simulink model "ID_Simulator"  (R2017b)
settings: Solver=VariableStepAuto  StartTime=0  StopTime=12  FixedStep=0.0005  EnableMultiTasking=on
InitFcn:
  | isSim = 1;
  | PreFunctions.CustomInitFcn;
  | PreFunctions.simulationInitFcn
values from neighbouring files (symbols this model uses):
  s = 0    [state_estimation.m]
undefined symbols (not defined in the file or in its folder): DiagnosticCodes, fcut_velocity_joint, GaitLibrary, motorPositions, motorVelocities, pelvisPosition, pelvisVelocity, UserParams, X, Y, Z
libraries: sm_lib x112, nesl_utility x20, ComponentLibrary x15, Contact_Forces_Lib x4, slrtlib x1, simulink x1, func_block_library x1
(part 1 of 5)
settings Model: Creator=case  LastModifiedBy=guoro
settings SolverCC: ZeroCrossControl=DisableAll  InsertRTBMode=Always
settings DataIOCC: SaveFormat=Array  SaveOutput=off  SaveState=on  DSMLogging=off
settings OptimizationCC: DefaultParameterBehavior=Inlined  UseFloatMulNetSlope=on  InlineInvariantSignals=on  EfficientFloat2IntCast=on  LifeSpan=inf  SimCompilerOptimization=on  AccelVerboseBuild=on
settings DebuggingCC: ReadBeforeWriteMsg=DisableAll  WriteAfterWriteMsg=DisableAll  WriteAfterReadMsg=DisableAll  ParameterUnderflowMsg=error  ParameterTunabilityLossMsg=error  UniqueDataStoreMsg=error  AllowSymbolicDim=off  StrictBusMsg=ErrorOnBusTreatedAsVector  SFUnexpectedBacktrackingDiag=warning  SFNoUnconditionalDefaultTransitionDiag=warning  SFExecutionAtInitializationDiag=none
settings HardwareCC: TargetBitPerPointer=64  TargetBitPerSizeT=64  TargetBitPerPtrDiffT=64  TargetLongLongMode=on  TargetIntDivRoundTo=Zero  TargetEndianess=LittleEndian  TargetWordSize=64  TargetHWDeviceType=MATLAB Host  ProdEqTarget=off
settings ModelReferenceCC: EnableParallelModelReferenceBuilds=on  ModelReferenceNumInstancesAllowed=Zero  ModelReferenceMinAlgLoopOccurrences=on  PropagateSignalLabelsOutOfModel=off
settings SFSimCC: SimUserIncludeDirs=gen\kin\src
settings SFSimCC: SimUserSources=|
  | ComPosition_src.c
  | ComVelocity_src.c
  | J_LeftToeBottomBack_src.c
  | J_LeftToeBottomFront_src.c
  | J_LeftToeBottom_src.c
  | J_LeftToeJoint_src.c
  | J_RightToeBottomBack_src.c
  | J_RightToeBottomFront_src.c
  | J_RightToeBottom_src.c
  | J_RightToeJoint_src.c
  | LeftToeBottomBack_src.c
  | LeftToeBottomFront_src.c
  | LeftToeBottom_src.c
  | LeftToeJoint_src.c
  | RightToeBottomBack_src.c
  | RightToeBottomFront_src.c
  | RightToeBottom_src.c
  | RightToeJoint_src.c
settings RTWCC: Description=Generic Real-Time Target  RTWUseSimCustomCode=on  CustomInclude=gen\kin\src  BuildConfiguration=Faster Runs  CheckMdlBeforeBuild=Warning
settings RTWCC: CustomSource=|
  | ComPosition_src.c
  | ComVelocity_src.c
  | J_LeftToeBottomBack_src.c
  | J_LeftToeBottomFront_src.c
  | J_LeftToeBottom_src.c
  | J_LeftToeJoint_src.c
  | J_RightToeBottomBack_src.c
  | J_RightToeBottomFront_src.c
  | J_RightToeBottom_src.c
  | J_RightToeJoint_src.c
  | LeftToeBottomBack_src.c
  | LeftToeBottomFront_src.c
  | LeftToeBottom_src.c
  | LeftToeJoint_src.c
  | RightToeBottomBack_src.c
  | RightToeBottomFront_src.c
  | RightToeBottom_src.c
  | RightToeJoint_src.c
settings CodeAppCC: GenerateComments=off  SimulinkBlockComments=off
settings GRTTargetCC: MatFileLogging=off  MultiInstanceERTCode=on  CodeInterfacePackaging=Reusable function  SupportNonFinite=off  GenerateAllocFcn=on
settings ConfigComp: CovMetricSettings=dw  CovHtmlReporting=on  CovSaveCumulativeToWorkspaceVar=on  CovSaveSingleToWorkspaceVar=on  CovExternalEMLEnable=off
settings SimscapeCC: SimscapeNormalizeSystem=off  SimscapeLogType=all  SimscapeLogSimulationStatistics=on  SimscapeLogOpenViewer=on  SimscapeLogLimitData=off  SimscapeLogDataHistory=40000
settings DiagnosticsConfigSet: SimMechanicsRigidlyBoundBlock=warning
settings ExplorerConfigSet: InternalSimMechanicsExplorerSettings="<ExplorerConfiguration><canonicalview>default</canonicalview><AnimationSetting><BasePlaybackSpeed>1.0</BasePlaybackSpeed><PlaybackSpeedFactor>1.0</PlaybackSpeedFactor></AnimationSetting><TilePanel><TileInfo><Tiles Columns=\"1\" Count=\"1\" Rows=\"1\"><Column Weight=\"1\"/><Row Weight=\"1\"/><Tile Height=\"1\" Width=\"1\" X=\"0\" Y=\"0\"/></Tiles></TileInfo><SceneInfo><SceneViewer><BGColor><R>0.60000002384185791</R><G>0.60000002384185791</G><B>0.60000002384185791</B></BGColor><Camera><DoPerspective>on</DoPerspective><Position><X>1.49424103443841916</X><Y>-1.5003618867302666</Y><Z>-0.448846928440659099</Z></Position><Center><X>-0.00575896556158084216</X><Y>-0.000361886730266602896</Y><Z>-0.948846928440659099</Z></Center><Up><X>0</X><Y>0</Y><Z>1</Z></Up><ViewLimDist>1</ViewLimDist><YLim>0.466307658154998583</YLim><XLim>2.07568807125632082</XLim></Camera></SceneViewer></SceneInfo></TilePanel><MechEditorPanel><Cameras><Camera><Id>Camera1</Id><Value><Name>Tracking Camera</Name><NativeCamera><PositionTrackingFeature>Cassie.Cassie_Simulation.World.Tracking_Camera.F</PositionTrackingFeature><CenterTrackingFeature>Cassie.Cassie_Simulation.World.Tracking_Camera_Target.F</CenterTrackingFeature><UpVectorTrackingFeature>Cassie.Cassie_Simulation.World.Tracking_Camera_Target.F</UpVectorTrackingFeature><CenterTrackingOrigin>on</CenterTrackingOrigin><UpVectorTrackingDirection>+Z</UpVectorTrackingDirection></NativeCamera></Value></Camera><Camera><Id>Camera2</Id><Value><Name>Fixed Camera</Name><NativeCamera><PositionTrackingFeature>Cassie.Cassie_Simulation.World.Fixed_Camera.F</PositionTrackingFeature><CenterTrackingFeature>Cassie.Cassie_Simulation.World.Fixed_Camera_Target.F</CenterTrackingFeature><UpVectorTrackingFeature>Cassie.Cassie_Simulation.World.Fixed_Camera_Target.F</UpVectorTrackingFeature><CenterTrackingOrigin>on</CenterTrackingOrigin><UpVectorTrackingDirection>+Z</UpVectorTrackingDirection></NativeCamera></Value></Camera></Cameras><GfxPanelCameraMap><MapElement CameraMLId=\"Camera1\" GfxPanelIndex=\"0\"/></GfxPanelCameraMap><VideoCreator><PlaybackSpeedRatio>1.0</PlaybackSpeedRatio><FrameRate>30</FrameRate><VideoFormat>Motion JPEG AVI</VideoFormat><FrameSize>auto</FrameSize></VideoCreator></MechEditorPanel></ExplorerConfiguration>"

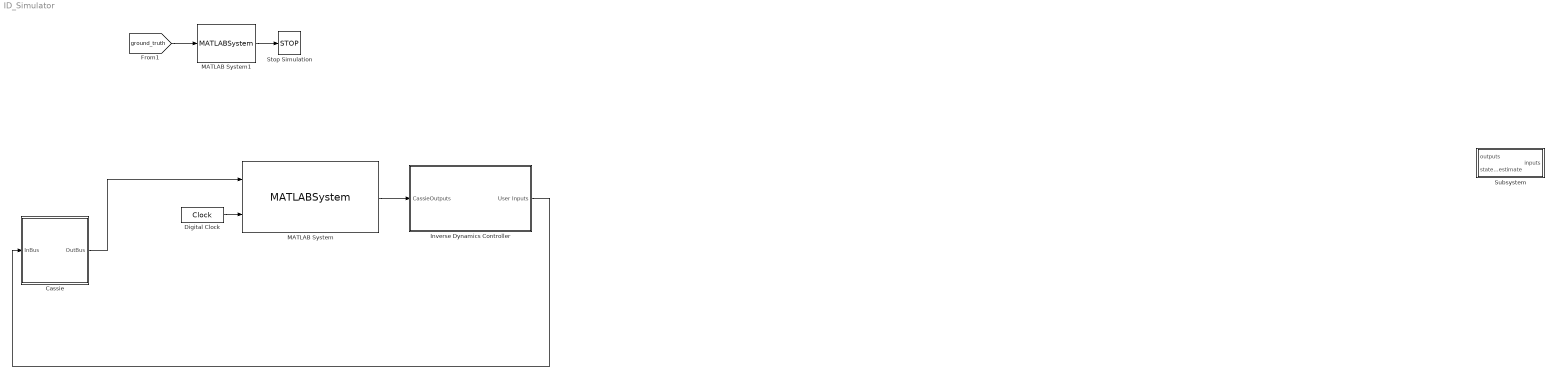
== system ID_Simulator ==
  Cassie : Subsystem  InitFcn=|  StartFcn=|  StopFcn=|
      InitFcn=|
      | % Start clock at initialization (used for computing real time performance)
      | initTime = tic;
      | 
      | % Import bus definitions
      | CassieModule.importBuses;
      StartFcn=|
      | % Store build time
      | buildTime = toc(initTime);
      StopFcn=|
      | % Store computation time
      | computationTime = toc(initTime) - buildTime;
      | 
      | % Get simulation time
      | simulationTime = get_param(bdroot, 'SimulationTime');
      | 
      | % Compute real time performance
      | percentRealTime = 100*simulationTime/computationTime;
      | 
      | % Display
      | fprintf('Build time: %0.2f seconds \n', buildTime);
      | fprintf('Simulation time: %0.2f seconds \n', simulationTime);
      | fprintf('Computation time: %0.2f seconds \n', computationTime);
      | fprintf('Performance: %0.2f%% real time \n', percentRealTime);
      mask Display: image('Cassie.png');
  Digital Clock : DigitalClock  SampleTime=UserParams.SampleTime
  Inverse Dynamics Controller : Subsystem
  MATLAB System : MATLABSystem  System=RemoteSpoofer  SimulateUsing=Code generation
      mask Type: RemoteSpoofer
      mask Display:
      | disp('RemoteSpoofer');
      | port_label('input',1,'cassieOutputs');
      | port_label('input',2,'t');
      | port_label('output',1,'cassieOutputs');
  MATLAB System1 : MATLABSystem  System=Stop_Criterion  SimulateUsing=Code generation
      mask Type: Stop_Criterion
      mask Display:
      | disp('Stop_Criterion');
      | port_label('input',1,'t');
      | port_label('output',1,'y');
  Stop Simulation : Stop
  Subsystem : Subsystem  AncestorBlock=FG_Controller_Library/Subsystem
  wires:
  Digital Clock/1 -> MATLAB System/2
  MATLAB System1/1 -> Stop Simulation/1
  [ground_truth] -> MATLAB System1/1
  Cassie/1(OutBus) -> MATLAB System/1
  Inverse Dynamics Controller/1(User Inputs) -> Cassie/1(InBus)
  MATLAB System/1 -> Inverse Dynamics Controller/1(CassieOutputs)

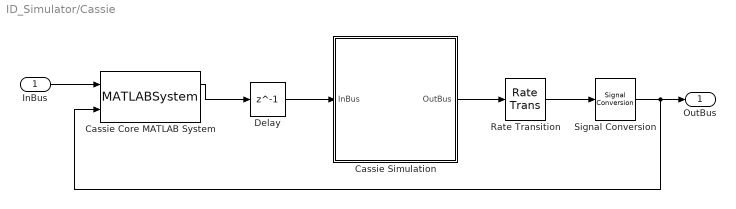
== system ID_Simulator/Cassie ==
  InBus : Inport  OutDataTypeStr=Bus: CassieUserInBus
  Cassie Core MATLAB System : MATLABSystem  System=CassieCoreSim  SimulateUsing=Code generation
      mask Type: CassieCoreSim
      mask Display: disp('CassieCoreSim');
  Cassie Simulation : Subsystem
      mask Display: image('Cassie.png');
  Delay : Delay  DelayLength=1
  Rate Transition : RateTransition  OutPortSampleTime=0.0005
  Signal Conversion : SignalConversion  ConversionOutput=Nonvirtual bus  OutDataTypeStr=Bus: CassieOutBus  OverrideOpt=off
  OutBus : Outport  OutDataTypeStr=Bus: CassieOutBus
  wires:
  Signal Conversion/1 -> OutBus/1, Cassie Core MATLAB System/2
  Cassie Simulation/1(OutBus) -> Rate Transition/1
  Rate Transition/1 -> Signal Conversion/1
  Delay/1 -> Cassie Simulation/1(InBus)
  Cassie Core MATLAB System/1 -> Delay/1
  InBus/1 -> Cassie Core MATLAB System/1

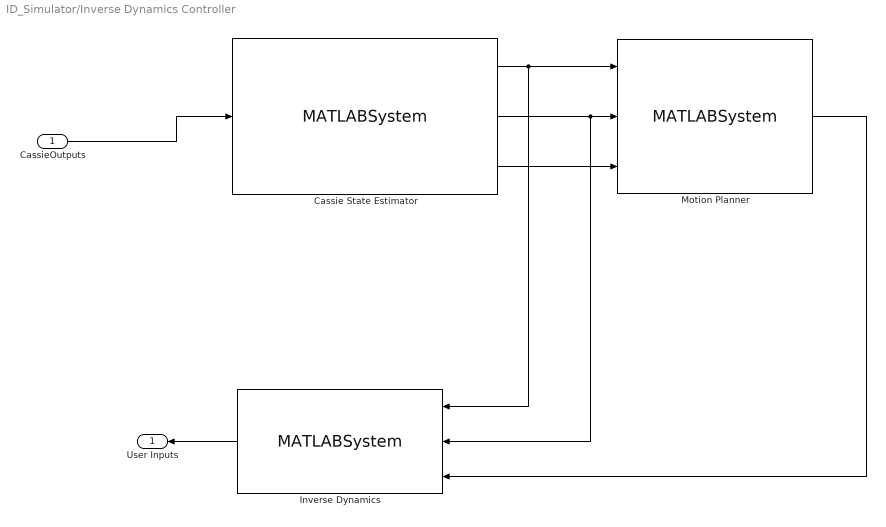
== system ID_Simulator/Inverse Dynamics Controller ==
  CassieOutputs : Inport
  Cassie State Estimator : MATLABSystem  System=stateEstimator  SimulateUsing=Code generation
      mask Type: stateEstimator
      mask Display:
      | disp('stateEstimator');
      | port_label('input',1,'cassieOutputs');
      | port_label('output',1,'q_fil');
      | port_label('output',2,'dq_fil');
      | port_label('output',3,'RadioButton');
  Inverse Dynamics : MATLABSystem  System=inverseDynamics  SimulateUsing=Code generation
      mask Type: inverseDynamics
      mask Display:
      | disp('inverseDynamics');
      | port_label('input',1,'q_fil');
      | port_label('input',2,'dq_fil');
      | port_label('input',3,'ddq_desired');
      | port_label('output',1,'userInputs');
  Motion Planner : MATLABSystem  System=motionPlanner  SimulateUsing=Code generation
      mask Type: motionPlanner
      mask Display:
      | disp('motionPlanner');
      | port_label('input',1,'q_fil');
      | port_label('input',2,'dq_fil');
      | port_label('input',3,'RadioButton');
      | port_label('output',1,'ddq_desired');
  User Inputs : Outport
  wires:
  CassieOutputs/1 -> Cassie State Estimator/1
  Motion Planner/1 -> Inverse Dynamics/3
  Cassie State Estimator/1 -> Inverse Dynamics/1, Motion Planner/1
  Cassie State Estimator/2 -> Inverse Dynamics/2, Motion Planner/2
  Cassie State Estimator/3 -> Motion Planner/3
  Inverse Dynamics/1 -> User Inputs/1

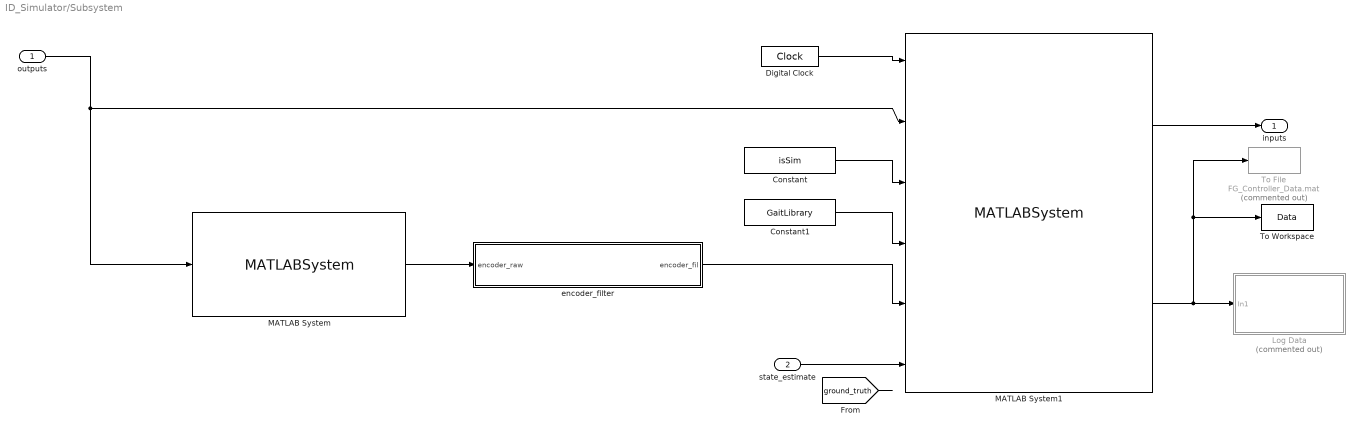
== system ID_Simulator/Subsystem ==
  outputs : Inport  OutDataTypeStr=Bus: CassieOutBus
  "state_estimate " : Inport  Port=2  OutDataTypeStr=double
  Constant : Constant  Value=isSim  OutDataTypeStr=boolean  LockScale=on
  Constant1 : Constant  Value=GaitLibrary  OutDataTypeStr=Bus: cassieGaitLibraryBus  LockScale=on
  Digital Clock : DigitalClock  SampleTime=UserParams.SampleTime
  Log Data : Subsystem  Commented=on
  MATLAB System : MATLABSystem  System=ExtractJointPosition  SimulateUsing=Code generation
      mask Type: ExtractJointPosition
      mask Display:
      | disp('ExtractJointPosition');
      | port_label('input',1,'cassieOutputs');
      | port_label('output',1,'JointPosition');
  MATLAB System1 : MATLABSystem  System=FG_Controller  Kp_pitch=c_Kp_pitch  Kd_pitch=c_Kd_pitch  Kp_roll=c_Kp_roll  Kd_roll=c_Kd_roll  Kp_yaw=c_Kp_yaw  Kd_yaw=c_Kd_yaw  Kp_abduction=c_Kp_abduction  Kp_rotation=c_Kp_rotation  Kp_thigh=c_Kp_thigh  Kp_knee=c_Kp_knee  Kp_toe=c_Kp_toe  Kd_abduction=c_Kd_abduction  Kd_rotation=c_Kd_rotation  Kd_thigh=c_Kd_thigh  Kd_knee=c_Kd_knee  Kd_toe=c_Kd_toe  Kfs_p=c_Kfs_p  Kfl_p=c_Kfl_p  Kfs_d=c_Kfs_d  Kfl_d=c_Kfl_d  Kp_toe_stand=c_Kp_toe_stand  Kd_toe_stand=c_Kd_toe_stand  Kp_lateral_stand=c_Kp_lateral_stand  Kd_lateral_stand=c_Kd_lateral_stand  Kp_abduction_stand=c_Kp_abduction_stand  Kd_abduction_stand=c_Kd_abduction_stand  Kp_thigh_stand=c_Kp_thigh_stand  Kd_thigh_stand=c_Kd_thigh_stand  Kp_knee_stand=c_Kp_knee_stand  Kd_knee_stand=c_Kd_knee_stand  Kp_rotation_stand=c_Kp_rotation_stand  Kd_rotation_stand=c_Kd_rotation_stand  fil_para_x=c_fil_para_x  fil_para_y=c_fil_para_y  stance_thre_ub=c_stance_thre_ub  stance_thre_lb=c_stance_thre_lb  lateral_velocity_weight=c_lateral_velocity_weight  init_lateral_velocity=c_init_lateral_velocity  abduction_inward_gain=c_abduction_inward_gain  joint_filter_choice=c_joint_filter_choice  shift_time=c_shift_time  shift_distance=c_shift_distance  standing_switch_time=c_standing_switch_time  toe_tilt_angle=c_toe_tilt_angle  final_sw_abduction=c_final_sw_abduction  final_st_abduction=c_final_st_abduction  pre_final_sw_abduction=c_pre_final_sw_abduction  sagittal_offset_exp=c_sagittal_offset_exp  lateral_offset_exp=c_lateral_offset_exp  turning_offset_exp=c_turning_offset_exp  stand_offset_exp=c_stand_offset_exp  u_abduction_cp=c_u_abduction_cp  u_abduction_swing_cp=c_u_abduction_swing_cp  u_thigh_cp=c_u_thigh_cp  u_knee_cp=c_u_knee_cp  fil_para_2=c_fil_para_2  fil_para_3=c_fil_para_3  fil_para_4=c_fil_para_4  fil_para_5=c_fil_para_5  force_step_end_s=c_force_step_end_s  SimulateUsing=Code generation
      mask Type: FG_Controller
      mask Display:
      | disp('FG_Controller');
      | port_label('input',1,'t');
      | port_label('input',2,'cassieOutputs');
      | port_label('input',3,'isSim');
      | port_label('input',4,'GaitLibrary');
      | port_label('input',5,'encoder_fil');
      | port_label('input',6,'state_estimation');
      | port_label('output',1,'userInputs');
      | port_label('output',2,'Data');
  To File : ToFile  Commented=on  Filename=FG_Controller_Data.mat  SaveFormat=Timeseries
  To Workspace : ToWorkspace  VariableName=Data  SaveFormat=Timeseries  SampleTime=-1
  encoder_filter : Subsystem  TreatAsAtomicUnit=on
  "inputs " : Outport
  wires:
  "state_estimate "/1 -> MATLAB System1/6
  outputs/1 -> MATLAB System/1, MATLAB System1/2
  Constant1/1 -> MATLAB System1/4
  Constant/1 -> MATLAB System1/3
  Digital Clock/1 -> MATLAB System1/1
  MATLAB System1/2 -> Log Data/1(In1), To Workspace/1, To File/1
  MATLAB System1/1 -> "inputs "/1
  encoder_filter/1(encoder_fil) -> MATLAB System1/5
  MATLAB System/1 -> encoder_filter/1(encoder_raw)
  [ground_truth] -> ?

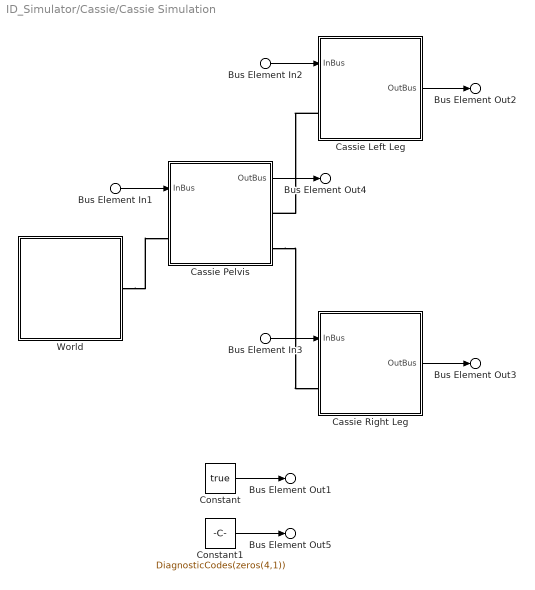
== system ID_Simulator/Cassie/Cassie Simulation ==
  Bus Element In2 : Inport  PortName=InBus  Element=leftLeg
  Bus Element In3 : Inport  PortName=InBus  Element=rightLeg
  Bus Element In1 : Inport  PortName=InBus  Element=pelvis
  Cassie Left Leg : Subsystem  AncestorBlock=CassieLibrary/Simulation/Cassie Leg  mask{config=Left, motorPositions=motorPositions(1:5), motorVelocities=motorVelocities(1:5)}
      mask prompts: config "Configuration:"; motorPositions "Initial Motor Positions (rad):"; motorVelocities "Initial Motor Velocities (rad/s):"
      mask init:
      | d = CassieDescriptor;
      | bodyIndex = @(s, name) find(arrayfun(@(s) isequal(s.name, name), s));
      | 
      | switch config
      |   case 1 % Left
      |     % Hip Roll
      |     b = d(bodyIndex(d, 'left-hip-roll'));
      |     set_param([gcb, '/Hip Roll Solid'], 'ExtGeomFileName', [b.name '.stl']);
      |     set_param([gcb, '/Hip Roll Solid'], 'Mass', mat2str(b.m));
      |     set_param([gcb, '/Hip Roll Solid'], 'CenterOfMass', mat2str(b.c));
      |     set_param([gcb, '/Hip Roll Solid'], 'MomentsOfInertia', mat2str(b.Ic(1:3)));
      |     set_param([gcb, '/Hip Roll Solid'], 'ProductsOfInertia', mat2str(b.Ic(4:6)));
      |     %set_param([gcb, '/Pelvis to Hip Roll'], 'TranslationCartesianOffset', mat2str(b.r));
      |     %set_param([gcb, '/Pelvis to Hip Roll'], 'RotationMatrix', mat2str(b.R));
      |     
      |     % Hip Yaw
      |     b = d(bodyIndex(d, 'left-hip-yaw'));
      |     set_param([gcb, '/Hip Yaw Solid'], 'ExtGeomFileName', [b.name '.stl']);
      |     set_param([gcb, '/Hip Yaw Solid'], 'Mass', mat2str(b.m));
      |     set_param([gcb, '/Hip Yaw Solid'], 'CenterOfMass', mat2str(b.c));
      |     set_param([gcb, '/Hip Yaw Solid'], 'MomentsOfInertia', mat2str(b.Ic(1:3)));
      |     set_param([gcb, '/Hip Yaw Solid'], 'ProductsOfInertia', mat2str(b.Ic(4:6)));
      |     set_param([gcb, '/Hip Roll to Hip Yaw'], 'TranslationCartesianOffset', mat2str(b.r));
      |     set_param([gcb, '/Hip Roll to Hip Yaw'], 'RotationMatrix', mat2str(b.R));
      |     
      |     % Hip Pitch
      |     b = d(bodyIndex(d, 'left-hip-pitch'));
      |     set_param([gcb, '/Hip Pitch Solid'], 'ExtGeomFileName', [b.name '.stl']);
      |     set_param([gcb, '/Hip Pitch Solid'], 'Mass', mat2str(b.m));
      |     set_param([gcb, '/Hip Pitch Solid'], 'CenterOfMass', mat2str(b.c));
      |     set_param([gcb, '/Hip Pitch Solid'], 'MomentsOfInertia', mat2str(b.Ic(1:3)));
      |     set_param([gcb, '/Hip Pitch Solid'], 'ProductsOfInertia', mat2str(b.Ic(4:6)));
      |     set_param([gcb, '/Hip Yaw to Hip Pitch'], 'TranslationCartesianOffset', mat2str(b.r));
      |     set_param([gcb, '/Hip Yaw to Hip Pitch'], 'RotationMatrix', mat2str(b.R));
      |     
      |     % Achilles Rod
      |     b = d(bodyIndex(d, 'left-achilles-rod'));
      |     set_param([gcb, '/Achilles Rod Solid'], 'ExtGeomFileName', [b.name '.stl']);
      |     set_param([gcb, '/Achilles Rod Solid'], 'Mass', mat2str(b.m));
      |     set_param([gcb, '/Achilles Rod Solid'], 'CenterOfMass', mat2str(b.c));
      |     set_param([gcb, '/Achilles Rod Solid'], 'MomentsOfInertia', mat2str(b.Ic(1:3)));
      |     set_param([gcb, '/Achilles Rod Solid'], 'ProductsOfInertia', mat2str(b.Ic(4:6)));
      |     set_param([gcb, '/Hip Pitch to Achilles Rod'], 'TranslationCartesianOffset', mat2str(b.r));
      |     set_param([gcb, '/Hip Pitch to Achilles Rod'], 'RotationMatrix', mat2str(b.R));
      |     
      |     % Knee
      |     b = d(bodyIndex(d, 'left-knee'));
      |     set_param([gcb, '/Knee Solid'], 'ExtGeomFileName', [b.name '.stl']);
      |     set_param([gcb, '/Knee Solid'], 'Mass', mat2str(b.m));
      |     set_param([gcb, '/Knee Solid'], 'CenterOfMass', mat2str(b.c));
      |     set_param([gcb, '/Knee Solid'], 'MomentsOfInertia', mat2str(b.Ic(1:3)));
      |     set_param([gcb, '/Knee Solid'], 'ProductsOfInertia', mat2str(b.Ic(4:6)));
      |     set_param([gcb, '/Hip Pitch to Knee'], 'TranslationCartesianOffset', mat2str(b.r));
      |     set_param([gcb, '/Hip Pitch to Knee'], 'RotationMatrix', mat2str(b.R));
      |     
      |     % Knee Spring
      |     b = d(bodyIndex(d, 'left-knee-spring'));
      |     set_param([gcb, '/Knee Spring Solid'], 'ExtGeomFileName', [b.name '.stl']);
      |     set_param([gcb, '/Knee Spring Solid'], 'Mass', mat2str(b.m));
      |     set_param([gcb, '/Knee Spring Solid'], 'CenterOfMass', mat2str(b.c));
      |     set_param([gcb, '/Knee Spring Solid'], 'MomentsOfInertia', mat2str(b.Ic(1:3)));
      |     set_param([gcb, '/Knee Spring Solid'], 'ProductsOfInertia', mat2str(b.Ic(4:6)));
      |     set_param([gcb, '/Knee to Knee Spring'], 'TranslationCartesianOffset', mat2str(b.r));
      |     set_param([gcb, '/Knee to Knee Spring'], 'RotationMatrix', mat2str(b.R));
      |     
      |     % Shin
      |     b = d(bodyIndex(d, 'left-shin'));
      |     set_param([gcb, '/Shin Solid'], 'ExtGeomFileName', [b.name '.stl']);
      |     set_param([gcb, '/Shin Solid'], 'Mass', mat2str(b.m));
      |     set_param([gcb, '/Shin Solid'], 'CenterOfMass', mat2str(b.c));
      |     set_param([gcb, '/Shin Solid'], 'MomentsOfInertia', mat2str(b.Ic(1:3)));
      |     set_param([gcb, '/Shin Solid'], 'ProductsOfInertia', mat2str(b.Ic(4:6)));
      |     set_param([gcb, '/Knee to Shin'], 'TranslationCartesianOffset', mat2str(b.r));
      |     set_param([gcb, '/Knee to Shin'], 'RotationMatrix', mat2str(b.R));
      |     
      |     % Tarsus
      |     b = d(bodyIndex(d, 'left-tarsus'));
      |     set_param([gcb, '/Tarsus Solid'], 'ExtGeomFileName', [b.name '.stl']);
      |     set_param([gcb, '/Tarsus Solid'], 'Mass', mat2str(b.m));
      |     set_param([gcb, '/Tarsus Solid'], 'CenterOfMass', mat2str(b.c));
      |     set_param([gcb, '/Tarsus Solid'], 'MomentsOfInertia', mat2str(b.Ic(1:3)));
      |     set_param([gcb, '/Tarsus Solid'], 'ProductsOfInertia', mat2str(b.Ic(4:6)));
      |     set_param([gcb, '/Shin to Tarsus'], 'TranslationCartesianOffset', mat2str(b.r));
      |     set_param([gcb, '/Shin to Tarsus'], 'RotationMatrix', mat2str(b.R));
      |     
      |     % Heel Spring
      |     b = d(bodyIndex(d, 'left-heel-spring'));
      |     set_param([gcb, '/Heel Spring Solid'], 'ExtGeomFileName', [b.name '.stl']);
      |     set_param([gcb, '/Heel Spring Solid'], 'Mass', mat2str(b.m));
      |     set_param([gcb, '/Heel Spring Solid'], 'CenterOfMass', mat2str(b.c));
      |     set_param([gcb, '/Heel Spring Solid'], 'MomentsOfInertia', mat2str(b.Ic(1:3)));
      |     set_param([gcb, '/Heel Spring Solid'], 'ProductsOfInertia', mat2str(b.Ic(4:6)));
      |     set_param([gcb, '/Tarsus to Heel Spring'], 'TranslationCartesianOffset', mat2str(b.r));
      |     set_param([gcb, '/Tarsus to Heel Spring'], 'RotationMatrix', mat2str(b.R));
      |     
      |     % Foot Crank
      |     b = d(bodyIndex(d, 'left-foot-crank'));
      |     set_param([gcb, '/Foot Crank Solid'], 'ExtGeomFileName', [b.name '.stl']);
      |     set_param([gcb, '/Foot Crank Solid'], 'Mass', mat2str(b.m));
      |     set_param([gcb, '/Foot Crank Solid'], 'CenterOfMass', mat2str(b.c));
      |     set_param([gcb, '/Foot Crank Solid'], 'MomentsOfInertia', mat2str(b.Ic(1:3)));
      |     set_param([gcb, '/Foot Crank Solid'], 'ProductsOfInertia', mat2str(b.Ic(4:6)));
      |     set_param([gcb, '/Tarsus to Foot Crank'], 'TranslationCartesianOffset', mat2str(b.r));
      |     set_param([gcb, '/Tarsus to Foot Crank'], 'RotationMatrix', mat2str(b.R));
      |     
      |     % Plantar Rod
      |     b = d(bodyIndex(d, 'left-plantar-rod'));
      |     set_param([gcb, '/Plantar Rod Solid'], 'ExtGeomFileName', [b.name '.stl']);
      |     set_param([gcb, '/Plantar Rod Solid'], 'Mass', mat2str(b.m));
      |     set_param([gcb, '/Plantar Rod Solid'], 'CenterOfMass', mat2str(b.c));
      |     set_param([gcb, '/Plantar Rod Solid'], 'MomentsOfInertia', mat2str(b.Ic(1:3)));
      |     set_param([gcb, '/Plantar Rod Solid'], 'ProductsOfInertia', mat2str(b.Ic(4:6)));
      |     set_param([gcb, '/Foot Crank to Plantar Rod'], 'TranslationCartesianOffset', mat2str(b.r));
      |     set_param([gcb, '/Foot Crank to Plantar Rod'], 'RotationMatrix', mat2str(b.R));
      |     
      |     % Foot
      |     b = d(bodyIndex(d, 'left-foot'));
      |     set_param([gcb, '/Foot Solid'], 'ExtGeomFileName', [b.name '.stl']);
      |     set_param([gcb, '/Foot Solid'], 'Mass', mat2str(b.m));
      |     set_param([gcb, '/Foot Solid'], 'CenterOfMass', mat2str(b.c));
      |     set_param([gcb, '/Foot Solid'], 'MomentsOfInertia', mat2str(b.Ic(1:3)));
      |     set_param([gcb, '/Foot Solid'], 'ProductsOfInertia', mat2str(b.Ic(4:6)));
      |     set_param([gcb, '/Tarsus to Foot'], 'TranslationCartesianOffset', mat2str(b.r));
      |     set_param([gcb, '/Tarsus to Foot'], 'RotationMatrix', mat2str(b.R));
      |     
      |     % Foot Pin
      |     %b = d(bodyIndex(d, 'left-foot-pin'));
      |     set_param([gcb, '/Foot to Foot Pin'], 'TranslationCartesianOffset', mat2str([0.055 0 0.00776]));
      |     set_param([gcb, '/Foot to Foot Pin'], 'RotationMatrix', mat2str(eye(3)));
      |     
      |     % Midfoot
      |     %b = d(bodyIndex(d, 'left-mid-foot'));
      |     set_param([gcb, '/Foot to Midfoot'], 'TranslationCartesianOffset', mat2str([0.01762 0.05219 0]));
      |     set_param([gcb, '/Foot to Midfoot'], 'RotationMatrix', mat2str([-0.766044443118978 0 -0.642787609686539;0.642787609686539 0 -0.766044443118978;0 -1 0]));
      |     
      |   case 2 % Right
      |     % Hip Roll
      |     b = d(bodyIndex(d, 'right-hip-roll'));
      |     set_param([gcb, '/Hip Roll Solid'], 'ExtGeomFileName', [b.name '.stl']);
      |     set_param([gcb, '/Hip Roll Solid'], 'Mass', mat2str(b.m));
      |     set_param([gcb, '/Hip Roll Solid'], 'CenterOfMass', mat2str(b.c));
      |     set_param([gcb, '/Hip Roll Solid'], 'MomentsOfInertia', mat2str(b.Ic(1:3)));
      |     set_param([gcb, '/Hip Roll Solid'], 'ProductsOfInertia', mat2str(b.Ic(4:6)));
      |     %set_param([gcb, '/Pelvis to Hip Roll'], 'TranslationCartesianOffset', mat2str(b.r));
      |     %set_param([gcb, '/Pelvis to Hip Roll'], 'RotationMatrix', mat2str(b.R));
      |     
      |     % Hip Yaw
      |     b = d(bodyIndex(d, 'right-hip-yaw'));
      |     set_param([gcb, '/Hip Yaw Solid'], 'ExtGeomFileName', [b.name '.stl']);
      |     set_param([gcb, '/Hip Yaw Solid'], 'Mass', mat2str(b.m));
      |     set_param([gcb, '/Hip Yaw Solid'], 'CenterOfMass', mat2str(b.c));
      |     set_param([gcb, '/Hip Yaw Solid'], 'MomentsOfInertia', mat2str(b.Ic(1:3)));
      |     set_param([gcb, '/Hip Yaw Solid'], 'ProductsOfInertia', mat2str(b.Ic(4:6)));
      |     set_param([gcb, '/Hip Roll to Hip Yaw'], 'TranslationCartesianOffset', mat2str(b.r));
      |     set_param([gcb, '/Hip Roll to Hip Yaw'], 'RotationMatrix', mat2str(b.R));
      |     
      |     % Hip Pitch
      |     b = d(bodyIndex(d, 'right-hip-pitch'));
      |     set_param([gcb, '/Hip Pitch Solid'], 'ExtGeomFileName', [b.name '.stl']);
      |     set_param([gcb, '/Hip Pitch Solid'], 'Mass', mat2str(b.m));
      |     set_param([gcb, '/Hip Pitch Solid'], 'CenterOfMass', mat2str(b.c));
      |     set_param([gcb, '/Hip Pitch Solid'], 'MomentsOfInertia', mat2str(b.Ic(1:3)));
      |     set_param([gcb, '/Hip Pitch Solid'], 'ProductsOfInertia', mat2str(b.Ic(4:6)));
      |     set_param([gcb, '/Hip Yaw to Hip Pitch'], 'TranslationCartesianOffset', mat2str(b.r));
      |     set_param([gcb, '/Hip Yaw to Hip Pitch'], 'RotationMatrix', mat2str(b.R));
      |     
      |     % Achilles Rod
      |     b = d(bodyIndex(d, 'right-achilles-rod'));
      |     set_param([gcb, '/Achilles Rod Solid'], 'ExtGeomFileName', [b.name '.stl']);
      |     set_param([gcb, '/Achilles Rod Solid'], 'Mass', mat2str(b.m));
      |     set_param([gcb, '/Achilles Rod Solid'], 'CenterOfMass', mat2str(b.c));
      |     set_param([gcb, '/Achilles Rod Solid'], 'MomentsOfInertia', mat2str(b.Ic(1:3)));
      |     set_param([gcb, '/Achilles Rod Solid'], 'ProductsOfInertia', mat2str(b.Ic(4:6)));
      |     set_param([gcb, '/Hip Pitch to Achilles Rod'], 'TranslationCartesianOffset', mat2str(b.r));
      |     set_param([gcb, '/Hip Pitch to Achilles Rod'], 'RotationMatrix', mat2str(b.R));
      |     
      |     % Knee
      |     b = d(bodyIndex(d, 'right-knee'));
      |     set_param([gcb, '/Knee Solid'], 'ExtGeomFileName', [b.name '.stl']);
      |     set_param([gcb, '/Knee Solid'], 'Mass', mat2str(b.m));
      |     set_param([gcb, '/Knee Solid'], 'CenterOfMass', mat2str(b.c));
      |     set_param([gcb, '/Knee Solid'], 'MomentsOfInertia', mat2str(b.Ic(1:3)));
      |     set_param([gcb, '/Knee Solid'], 'ProductsOfInertia', mat2str(b.Ic(4:6)));
      |     set_param([gcb, '/Hip Pitch to Knee'], 'TranslationCartesianOffset', mat2str(b.r));
      |     set_param([gcb, '/Hip Pitch to Knee'], 'RotationMatrix', mat2str(b.R));
      |     
      |     % Knee Spring
      |     b = d(bodyIndex(d, 'right-knee-spring'));
      |     set_param([gcb, '/Knee Spring Solid'], 'ExtGeomFileName', [b.name '.stl']);
      |     set_param([gcb, '/Knee Spring Solid'], 'Mass', mat2str(b.m));
      |     set_param([gcb, '/Knee Spring Solid'], 'CenterOfMass', mat2str(b.c));
      |     set_param([gcb, '/Knee Spring Solid'], 'MomentsOfInertia', mat2str(b.Ic(1:3)));
      |     set_param([gcb, '/Knee Spring Solid'], 'ProductsOfInertia', mat2str(b.Ic(4:6)));
      |     set_param([gcb, '/Knee to Knee Spring'], 'TranslationCartesianOffset', mat2str(b.r));
      |     set_param([gcb, '/Knee to Knee Spring'], 'RotationMatrix', mat2str(b.R));
      |     
      |     % Shin
      |     b = d(bodyIndex(d, 'right-shin'));
      |     set_param([gcb, '/Shin Solid'], 'ExtGeomFileName', [b.name '.stl']);
      |     set_param([gcb, '/Shin Solid'], 'Mass', mat2str(b.m));
      |     set_param([gcb, '/Shin Solid'], 'CenterOfMass', mat2str(b.c));
      |     set_param([gcb, '/Shin Solid'], 'MomentsOfInertia', mat2str(b.Ic(1:3)));
      |     set_param([gcb, '/Shin Solid'], 'ProductsOfInertia', mat2str(b.Ic(4:6)));
      |     set_param([gcb, '/Knee to Shin'], 'TranslationCartesianOffset', mat2str(b.r));
      |     set_param([gcb, '/Knee to Shin'], 'RotationMatrix', mat2str(b.R));
      |     
      |     % Tarsus
      |     b = d(bodyIndex(d, 'right-tarsus'));
      |     set_param([gcb, '/Tarsus Solid'], 'ExtGeomFileName', [b.name '.stl']);
      |     set_param([gcb, '/Tarsus Solid'], 'Mass', mat2str(b.m));
      |     set_param([gcb, '/Tarsus Solid'], 'CenterOfMass', mat2str(b.c));
      |     set_param([gcb, '/Tarsus Solid'], 'MomentsOfInertia', mat2str(b.Ic(1:3)));
      |     set_param([gcb, '/Tarsus Solid'], 'ProductsOfInertia', mat2str(b.Ic(4:6)));
      |     set_param([gcb, '/Shin to Tarsus'], 'TranslationCartesianOffset', mat2str(b.r));
      |     set_param([gcb, '/Shin to Tarsus'], 'RotationMatrix', mat2str(b.R));
      |     
      |     % Heel Spring
      |     b = d(bodyIndex(d, 'right-heel-spring'));
      |     set_param([gcb, '/Heel Spring Solid'], 'ExtGeomFileName', [b.name '.stl']);
      |     set_param([gcb, '/Heel Spring Solid'], 'Mass', mat2str(b.m));
      |     set_param([gcb, '/Heel Spring Solid'], 'CenterOfMass', mat2str(b.c));
      |     set_param([gcb, '/Heel Spring Solid'], 'MomentsOfInertia', mat2str(b.Ic(1:3)));
      |     set_param([gcb, '/Heel Spring Solid'], 'ProductsOfInertia', mat2str(b.Ic(4:6)));
      |     set_param([gcb, '/Tarsus to Heel Spring'], 'TranslationCartesianOffset', mat2str(b.r));
      |     set_param([gcb, '/Tarsus to Heel Spring'], 'RotationMatrix', mat2str(b.R));
      |     
      |     % Foot Crank
      |     b = d(bodyIndex(d, 'right-foot-crank'));
      |     set_param([gcb, '/Foot Crank Solid'], 'ExtGeomFileName', [b.name '.stl']);
      |     set_param([gcb, '/Foot Crank Solid'], 'Mass', mat2str(b.m));
      |     set_param([gcb, '/Foot Crank Solid'], 'CenterOfMass', mat2str(b.c));
      |     set_param([gcb, '/Foot Crank Solid'], 'MomentsOfInertia', mat2str(b.Ic(1:3)));
      |     set_param([gcb, '/Foot Crank Solid'], 'ProductsOfInertia', mat2str(b.Ic(4:6)));
      |     set_param([gcb, '/Tarsus to Foot Crank'], 'TranslationCartesianOffset', mat2str(b.r));
      |     set_param([gcb, '/Tarsus to Foot Crank'], 'RotationMatrix', mat2str(b.R));
      |     
      |     % Plantar Rod
      |     b = d(bodyIndex(d, 'right-plantar-rod'));
      |     set_param([gcb, '/Plantar Rod Solid'], 'ExtGeomFileName', [b.name '.stl']);
      |     set_param([gcb, '/Plantar Rod Solid'], 'Mass', mat2str(b.m));
      |     set_param([gcb, '/Plantar Rod Solid'], 'CenterOfMass', mat2str(b.c));
      |     set_param([gcb, '/Plantar Rod Solid'], 'MomentsOfInertia', mat2str(b.Ic(1:3)));
      |     set_param([gcb, '/Plantar Rod Solid'], 'ProductsOfInertia', mat2str(b.Ic(4:6)));
      |     set_param([gcb, '/Foot Crank to Plantar Rod'], 'TranslationCartesianOffset', mat2str(b.r));
      |     set_param([gcb, '/Foot Crank to Plantar Rod'], 'RotationMatrix', mat2str(b.R));
      |     
      |     % Foot
      |     b = d(bodyIndex(d, 'right-foot'));
      |     set_param([gcb, '/Foot Solid'], 'ExtGeomFileName', [b.name '.stl']);
      |     set_param([gcb, '/Foot Solid'], 'Mass', mat2str(b.m));
      |     set_param([gcb, '/Foot Solid'], 'CenterOfMass', mat2str(b.c));
      |     set_param([gcb, '/Foot Solid'], 'MomentsOfInertia', mat2str(b.Ic(1:3)));
      |     set_param([gcb, '/Foot Solid'], 'ProductsOfInertia', mat2str(b.Ic(4:6)));
      |     set_param([gcb, '/Tarsus to Foot'], 'TranslationCartesianOffset', mat2str(b.r));
      |     set_param([gcb, '/Tarsus to Foot'], 'RotationMatrix', mat2str(b.R));
      |     
      |     % Foot Pin
      |     %b = d(bodyIndex(d, 'right-foot-pin'));
      |     set_param([gcb, '/Foot to Foot Pin'], 'TranslationCartesianOffset', mat2str([0.055 0 -0.00776]));
      |     set_param([gcb, '/Foot to Foot Pin'], 'RotationMatrix', mat2str(eye(3)));
      |     
      |     % Midfoot
      |     %b = d(bodyIndex(d, 'right-mid-foot'));
      |     set_param([gcb, '/Foot to Midfoot'], 'TranslationCartesianOffset', mat2str([0.01762 0.05219 0]));
      |     set_param([gcb, '/Foot to Midfoot'], 'RotationMatrix', mat2str([-0.766044443118978 0 -0.642787609686539;0.642787609686539 0 -0.766044443118978;0 -1 0]));
      | end % switch
      | 
      | % Check if block is not in library model
      | if ~bdIsLibrary(bdroot)
      |   % Construct discrete filter for velocity estimation
      |   dt = str2num(get_param(bdroot, 'FixedStep'));
      |   filter1 = ButterworthFilter(2);
      |   filter1.setTimeConstant(0.003, dt);
      |   filter2 = BackwardDifferencingFilter(2);
      |   filter2.setSampleTime(dt);
      |   filter3 = Filter(filter1, filter2, 'cascade');
      |   [a, b] = filter3.getCoefficients;
      |   
      |   % Set discrete filter coefficients    
      |   set_param([gcb '/Shin Filter'], 'a', mat2str(a));
      |   set_param([gcb '/Shin Filter'], 'b', mat2str(b));
      |   set_param([gcb '/Tarsus Filter'], 'a', mat2str(a));
      |   set_param([gcb '/Tarsus Filter'], 'b', mat2str(b));
      |   set_param([gcb '/Foot Filter'], 'a', mat2str(a));
      |   set_param([gcb '/Foot Filter'], 'b', mat2str(b));
      | end % if
      mask TypeOptions config: Left | Right
  Cassie Pelvis : Subsystem
  Cassie Right Leg : Subsystem  AncestorBlock=CassieLibrary/Simulation/Cassie Leg  mask{config=Right, motorPositions=motorPositions(6:10), motorVelocities=motorVelocities(6:10)}
      mask prompts: config "Configuration:"; motorPositions "Initial Motor Positions (rad):"; motorVelocities "Initial Motor Velocities (rad/s):"
      mask init: same as ID_Simulator/Cassie/Cassie Simulation/Cassie Left Leg
      mask TypeOptions config: Left | Right
  Constant : Constant  Value=true
  Constant1 : Constant  Value=DiagnosticCodes(zeros(4,1))
  World : Subsystem  AncestorBlock=ComponentLibrary/Simulation/World
  Bus Element Out4 : Outport  PortName=OutBus  Element=pelvis
  Bus Element Out2 : Outport  PortName=OutBus  Element=leftLeg
  Bus Element Out3 : Outport  PortName=OutBus  Element=rightLeg
  Bus Element Out1 : Outport  PortName=OutBus  Element=isCalibrated
  Bus Element Out5 : Outport  PortName=OutBus  Element=messages
  wires:
  Constant1/1 -> Bus Element Out5/1
  Constant/1 -> Bus Element Out1/1
  Bus Element In1/1 -> Cassie Pelvis/1(InBus)
  Cassie Right Leg/1(OutBus) -> Bus Element Out3/1
  Bus Element In2/1 -> Cassie Left Leg/1(InBus)
  Cassie Left Leg/1(OutBus) -> Bus Element Out2/1
  Bus Element In3/1 -> Cassie Right Leg/1(InBus)
  Cassie Pelvis/1(OutBus) -> Bus Element Out4/1
  connections:
  World/RConn1 -- Cassie Pelvis/LConn1
  Cassie Left Leg/LConn1 -- Cassie Pelvis/RConn1
  Cassie Pelvis/RConn2 -- Cassie Right Leg/LConn1

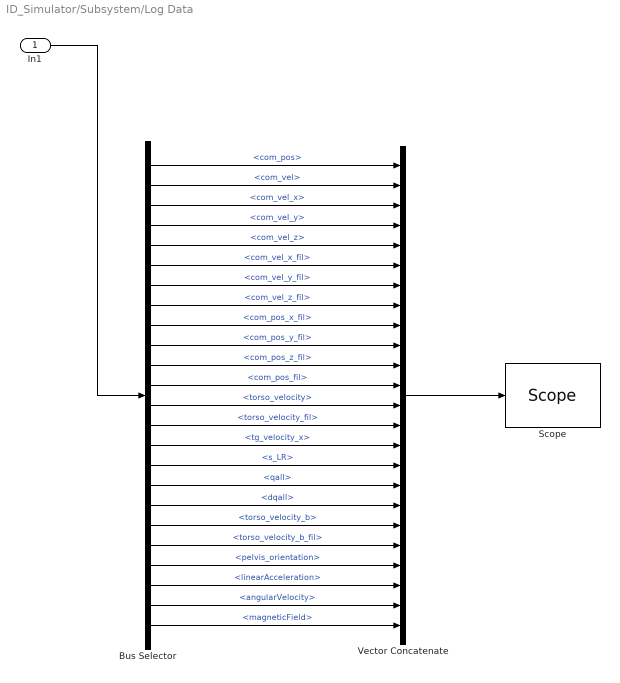
== system ID_Simulator/Subsystem/Log Data ==
  In1 : Inport  OutDataTypeStr=Bus: cassieDataBus
  Bus Selector : BusSelector  OutputSignals=com_pos,com_vel,com_vel_x,com_vel_y,com_vel_z,com_vel_x_fil,com_vel_y_fil,com_vel_z_fil,com_pos_x_fil,com_pos_y_fil,com_pos_z_fil,com_pos_fil,torso_velocity,torso_velocity_fil,tg_velocity_x,s_LR,qall,dqall,torso_velocity_b,torso_velocity_b_fil,pelvis_orientation,linearAcceleration,angularVelocity,magneticField
  "Scope " : slrtlib/Displays and Logging/Scope   scopeno=5  scopetype=File  autostart=on  viewmode=Graphical redraw  formatstr='%15.6f'  grid=on  ylimits=[0,0]  nosamples=250  noprepostsamples=0  interleave=1  triggermode=FreeRun  triggersignal=1  trigsignalfromport=off  triggerlevel=0.0  triggerslope=Either  triggerscope=1  triggersample=0  filename=data.dat  mode=Lazy  writesize=512*8  autorestart=on  dynamicfilemode=off  maxwritefilesize=4*1024^3
  Vector Concatenate : Concatenate  NumInputs=24
  wires:
  Bus Selector/24 -> Vector Concatenate/24  "<magneticField>"
  Bus Selector/23 -> Vector Concatenate/23  "<angularVelocity>"
  Bus Selector/22 -> Vector Concatenate/22  "<linearAcceleration>"
  Bus Selector/21 -> Vector Concatenate/21  "<pelvis_orientation>"
  Bus Selector/20 -> Vector Concatenate/20  "<torso_velocity_b_fil>"
  Bus Selector/19 -> Vector Concatenate/19  "<torso_velocity_b>"
  Bus Selector/18 -> Vector Concatenate/18  "<dqall>"
  Bus Selector/17 -> Vector Concatenate/17  "<qall>"
  Bus Selector/16 -> Vector Concatenate/16  "<s_LR>"
  In1/1 -> Bus Selector/1
  Vector Concatenate/1 -> "Scope "/1
  Bus Selector/1 -> Vector Concatenate/1  "<com_pos>"
  Bus Selector/2 -> Vector Concatenate/2  "<com_vel>"
  Bus Selector/3 -> Vector Concatenate/3  "<com_vel_x>"
  Bus Selector/4 -> Vector Concatenate/4  "<com_vel_y>"
  Bus Selector/5 -> Vector Concatenate/5  "<com_vel_z>"
  Bus Selector/6 -> Vector Concatenate/6  "<com_vel_x_fil>"
  Bus Selector/7 -> Vector Concatenate/7  "<com_vel_y_fil>"
  Bus Selector/8 -> Vector Concatenate/8  "<com_vel_z_fil>"
  Bus Selector/9 -> Vector Concatenate/9  "<com_pos_x_fil>"
  Bus Selector/10 -> Vector Concatenate/10  "<com_pos_y_fil>"
  Bus Selector/11 -> Vector Concatenate/11  "<com_pos_z_fil>"
  Bus Selector/12 -> Vector Concatenate/12  "<com_pos_fil>"
  Bus Selector/13 -> Vector Concatenate/13  "<torso_velocity>"
  Bus Selector/14 -> Vector Concatenate/14  "<torso_velocity_fil>"
  Bus Selector/15 -> Vector Concatenate/15  "<tg_velocity_x>"

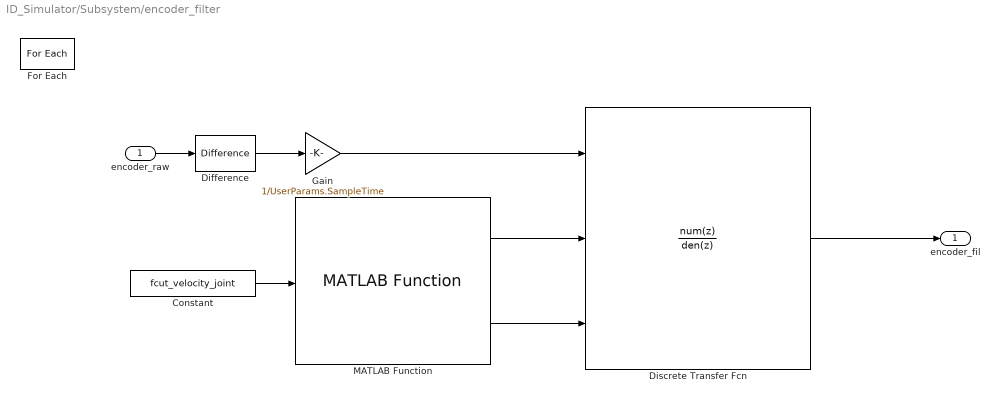
== system ID_Simulator/Subsystem/encoder_filter ==
  encoder_raw : Inport  Partition=on  PartitionDimension=1  PartitionWidth=1  PartitionOffset=0
  Constant : Constant  Value=fcut_velocity_joint
  Difference : simulink/Discrete/Difference  ICPrevInput=0.0  OutMin=[]  OutMax=[]  OutDataType=fixdt(1, 16)  OutScaling=2^-10  DoSatur=off
  Discrete Transfer Fcn : DiscreteTransferFcn  NumeratorSource=Input port  DenominatorSource=Input port  SampleTime=UserParams.SampleTime  a0EqualsOne=on
      settings: InputPortMap=u0,p1,p3
  For Each : ForEach  DisableCoverage=on  IndexMode=One-based
  Gain : Gain  Gain=1/UserParams.SampleTime
  MATLAB Function : func_block_library/MATLAB Function
  encoder_fil : Outport  ConcatenationDimension=1
  wires:
  MATLAB Function/2 -> Discrete Transfer Fcn/3
  MATLAB Function/1 -> Discrete Transfer Fcn/2
  Discrete Transfer Fcn/1 -> encoder_fil/1
  Gain/1 -> Discrete Transfer Fcn/1
  Difference/1 -> Gain/1
  Constant/1 -> MATLAB Function/1
  encoder_raw/1 -> Difference/1
